simulink model "motor_drive_control"  (R2022a)
settings: Solver=VariableStepAuto  StartTime=0.0  StopTime=10
undefined symbols (not defined in the file): g, J, k, Ke, kE, kF, kM, Ku, Kw, l, L, ml, n, pd, R
libraries: fuzblock x1
settings Model: Creator=clever0ne  LastModifiedBy=clever0ne
settings SolverCC: ZeroCrossAlgorithm=Adaptive
settings DataIOCC: SaveFormat=Array  ReturnWorkspaceOutputs=off
settings DebuggingCC: IgnoredZcDiagnostic=none

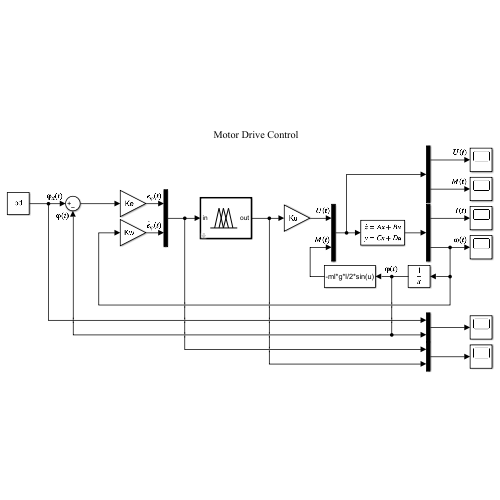
[thumbnail: Simulink's stored preview of the top-level diagram]
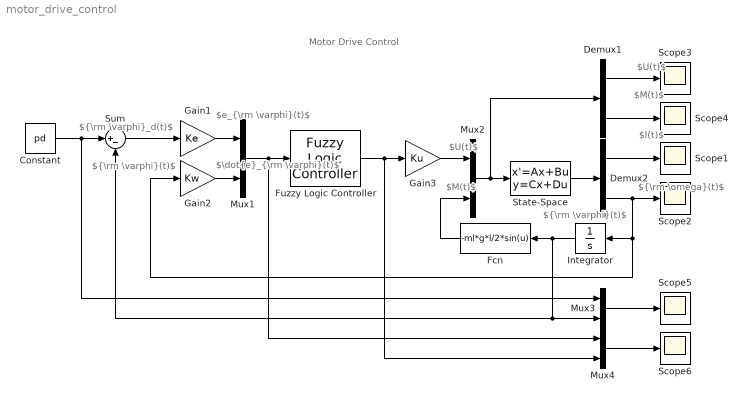
== system motor_drive_control ==
  note: $U(t)$
  note: Motor Drive Control
  note: $M(t)$
  note: $M(t)$
  note: $U(t)$
  note: $I(t)$
  note: ${\rm \omega}(t)$
  note: $e_{\rm \varphi}(t)$
  note: $\dot{e}_{\rm \varphi}(t)$
  note: ${\rm \varphi}(t)$
  note: ${\rm \varphi}(t)$
  note: ${\rm \varphi}_d(t)$
  Constant : Constant  Value=pd
  Demux1 : Demux  Outputs=2
  Demux2 : Demux  Outputs=2
  Fcn : Fcn  Expr=-ml*g*l/2*sin(u)
  Fuzzy Logic Controller : fuzblock/Fuzzy Logic  Controller  FIS=fis  OutputSampleNumber=101  DataType=double  FuzzifiedInputs=off  RuleFiringStrengths=off  RuleOutputs=off  AggregatedOutputs=off  SimulateUsing=Interpreted execution  OutOfRangeInputValueMessage=none  NoRuleFiredMessage=none  EmptyOutputFuzzySetMessage=none
  Gain1 : Gain  Gain=Ke
  Gain2 : Gain  Gain=Kw
  Gain3 : Gain  Gain=Ku
  Integrator : Integrator
  Mux{1..4} (4 alike) : Mux  Inputs=2
  Scope{1..6} (6 alike) : Scope
  State-Space : StateSpace  A=[-R/L, -k*kE/L; n*k*kM/J, -kF/J]  B=[1/L, 0; 0, 1/J]  C=eye(2)  D=zeros(2)  InitialCondition=0
  Sum : Sum  Inputs=|+-
  wires:
  State-Space/1 -> Demux2/1
  Demux2/1 -> Scope1/1
  Mux2/1 -> Demux1/1, State-Space/1
  Integrator/1 -> Mux3/2, Sum/2, Fcn/1
  Constant/1 -> Sum/1, Mux3/1
  Fcn/1 -> Mux2/2
  Sum/1 -> Gain1/1
  Demux2/2 -> Integrator/1, Gain2/1, Scope2/1
  Mux1/1 -> Fuzzy Logic Controller/1, Mux4/1
  Fuzzy Logic Controller/1 -> Gain3/1, Mux4/2
  Gain1/1 -> Mux1/1
  Gain2/1 -> Mux1/2
  Gain3/1 -> Mux2/1
  Mux3/1 -> Scope5/1
  Mux4/1 -> Scope6/1
  Demux1/2 -> Scope4/1
  Demux1/1 -> Scope3/1
